simulink model "sampleModel2035"  (R2023a)
settings: Solver=VariableStepAuto  StartTime=0.0  StopTime=10.0  RelTol=1e-3
libraries: hdlsllib x11, simulink x2
settings Model: Creator=user1  LastModifiedBy=user1

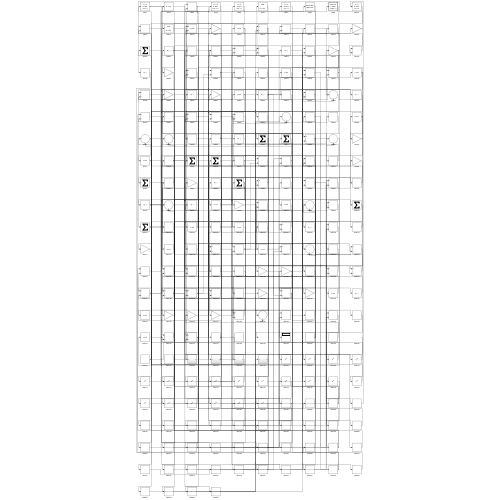
[thumbnail: Simulink's stored preview of the top-level diagram]
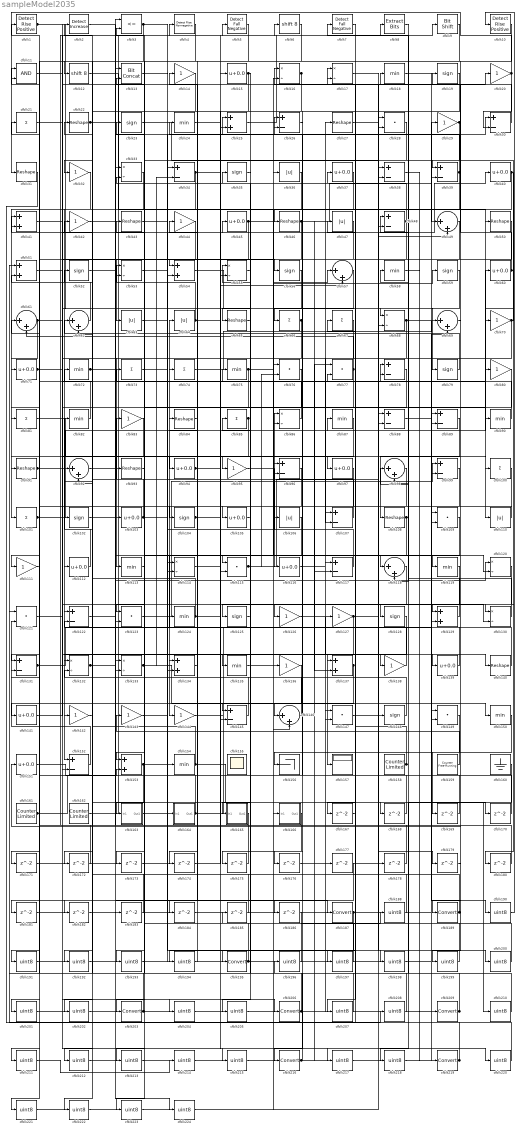
== system sampleModel2035 ==
  cfblk1 : hdlsllib/Logic and Bit Operations/Detect Rise Positive  vinit=0  OutDataTypeStr=boolean
  cfblk10 : hdlsllib/Logic and Bit Operations/Detect Rise Positive  vinit=0  OutDataTypeStr=boolean
  cfblk{21,66..67,73..74,81,85,100..101} (9 alike) : Sum  Inputs=+
  cfblk{19,23,35,52,56,59,79,102,104,125,128,148} (12 alike) : Signum
  cfblk{15,37,40,45,60,71,94,97,103,105,112,116,139,141,151} (15 alike) : Bias  Bias=0.0  SaturateOnIntegerOverflow=off
  cfblk{36,47,63..64,106,110} (6 alike) : Abs  SaturateOnIntegerOverflow=off
  cfblk{26,30,34,38..39,48,78,88..89,96,99,107,117,122,131,145,152} (17 alike) : Sum  Inputs=+-
  cfblk{22,27,31,43,46,50,65,84,91,93,108,140} (12 alike) : Reshape
  cfblk{28,76..77,109,115,121,123,147,149} (9 alike) : DotProduct  OutDataTypeStr=Inherit: Inherit via internal rule
  cfblk11 : Logic  AllPortsSameDT=off  OutDataTypeStr=boolean
  cfblk{14,20,29,32,42,44,70,80,83,95,111,126..127,136,138,142..144} (18 alike) : Gain
  cfblk{18,24,58,72,75,82,87,90,113,119,124,135,150,154} (14 alike) : MinMax
  cfblk{16..17,33,53,55,68,86,114,120,130,132..133} (12 alike) : Product  Inputs=*/  RndMeth=Zero  SaturateOnIntegerOverflow=on
  cfblk{49,57,61..62,69,92,98,118,146} (9 alike) : Sum  Inputs=|++
  cfblk12 : ArithShift  BitShiftNumber=8
  cfblk{25,41,51,54,129,134,137,153} (8 alike) : Sum
  cfblk13 : hdlsllib/Logic and Bit Operations/Bit Concat  numInputs=2
  cfblk155 : Scope
      settings: Floating=on
  cfblk156 : Terminator
  cfblk157 : Display
  cfblk158 : hdlsllib/Sources/Counter Limited  uplimit=7  tsamp=-1
  cfblk159 : hdlsllib/Sources/Counter Free-Running  NumBits=16  tsamp=-1
  cfblk160 : Ground
  cfblk161 : hdlsllib/Sources/Counter Limited  uplimit=7  tsamp=-1
  cfblk162 : hdlsllib/Sources/Counter Limited  uplimit=7  tsamp=-1
  cfblk163 : Subsystem
      settings: LibrarySourceBlock=|
      | hdlsllib/Ports &
      | Subsystems/Subsystem
  cfblk164 : Subsystem
      settings: LibrarySourceBlock=|
      | hdlsllib/Ports &
      | Subsystems/Subsystem
  cfblk165 : Subsystem
      settings: LibrarySourceBlock=|
      | hdlsllib/Ports &
      | Subsystems/Subsystem
  cfblk166 : Subsystem
      settings: LibrarySourceBlock=|
      | hdlsllib/Ports &
      | Subsystems/Subsystem
  cfblk{167..186} (20 alike) : Delay  SampleTime=1
  cfblk{187,189,195,203,206,209,216,219} (8 alike) : DataTypeConversion  SaturateOnIntegerOverflow=off  RndMeth=Floor
  cfblk{188,190..194,196..202,204..205,207..208,210..215,217..218,220..224} (30 alike) : DataTypeConversion  OutDataTypeStr=uint8  SaturateOnIntegerOverflow=off  RndMeth=Floor
  cfblk2 : simulink/Logic and Bit Operations/Detect Increase  vinit=0.0  OutDataTypeStr=boolean
      settings: LibrarySourceBlock=|
      | hdlsllib/Logic and Bit
      | Operations/Detect
      | Increase
  cfblk3 : RelationalOperator  Operator=<=  OutDataTypeStr=boolean  InputSameDT=off
  cfblk4 : hdlsllib/Logic and Bit Operations/Detect Rise Nonnegative  vinit=0  OutDataTypeStr=boolean
  cfblk5 : hdlsllib/Logic and Bit Operations/Detect Fall Negative  vinit=0  OutDataTypeStr=boolean
  cfblk6 : ArithShift  BitShiftNumber=8
  cfblk7 : hdlsllib/Logic and Bit Operations/Detect Fall Negative  vinit=0  OutDataTypeStr=boolean
  cfblk8 : simulink/Logic and Bit Operations/Extract Bits  bitsToExtract=Upper half  numBits=8  bitIdxRange=[0 7]  outScalingMode=Preserve fixed-point scaling
      settings: LibrarySourceBlock=|
      | hdlsllib/Logic and Bit
      | Operations/Extract Bits
  cfblk9 : hdlsllib/Logic and Bit Operations/Bit Shift  mode=Shift Left Logical  N=0
  wires:
  cfblk36/1 -> cfblk152/1
  cfblk117/1 -> cfblk86/1
  cfblk162/1 -> cfblk40/1
  cfblk165/1(Out1) -> cfblk4/1
  cfblk66/1 -> cfblk113/1, cfblk152/2
  cfblk72/1 -> cfblk5/1, cfblk119/1
  cfblk52/1 -> cfblk133/1
  cfblk118/1 -> cfblk128/1
  cfblk128/1 -> cfblk157/1
  cfblk103/1 -> cfblk83/1, cfblk130/2
  cfblk25/1 -> cfblk9/1
  cfblk75/1 -> cfblk123/1, cfblk57/1
  cfblk23/1 -> cfblk148/1
  cfblk124/1 -> cfblk92/2, cfblk217/1
  cfblk139/1 -> cfblk64/1
  cfblk59/1 -> cfblk79/1
  cfblk89/1 -> cfblk108/1
  cfblk123/1 -> cfblk99/1
  cfblk57/1 -> cfblk95/1
  cfblk20/1 -> cfblk31/1, cfblk30/2
  cfblk49/1 -> cfblk63/1
  cfblk1/1 -> cfblk68/1, cfblk68/2
  cfblk104/1 -> cfblk15/1, cfblk30/1
  cfblk13/1 -> cfblk164/1(In1)
  cfblk37/1 -> cfblk122/1
  cfblk38/1 -> cfblk219/1
  cfblk129/1 -> cfblk62/1
  cfblk146/1 -> cfblk52/1
  cfblk152/1 -> cfblk121/2
  cfblk86/1 -> cfblk43/1
  cfblk16/1 -> cfblk94/1, cfblk134/2
  cfblk142/1 -> cfblk42/1
  cfblk69/1 -> cfblk151/1
  cfblk32/1 -> cfblk101/1
  cfblk131/1 -> cfblk76/1, cfblk135/1
  cfblk2/1 -> cfblk187/1
  cfblk5/1 -> cfblk153/1
  cfblk26/1 -> cfblk46/1
  cfblk106/1 -> cfblk144/1
  cfblk42/1 -> cfblk19/1
  cfblk109/1 -> cfblk203/1
  cfblk10/1 -> cfblk189/1
  cfblk132/1 -> cfblk120/1, cfblk224/1
  cfblk100/1 -> cfblk142/1
  cfblk45/1 -> cfblk120/2, cfblk181/1
  cfblk154/1 -> cfblk92/1, cfblk210/1
  cfblk135/1 -> cfblk59/1
  cfblk107/1 -> cfblk41/1
  cfblk65/1 -> cfblk125/1
  cfblk164/1(Out1) -> cfblk89/1, cfblk21/1
  cfblk81/1 -> cfblk97/1
  cfblk40/1 -> cfblk86/2, cfblk70/1
  cfblk110/1 -> cfblk103/1
  cfblk77/1 -> cfblk126/1, cfblk61/2
  cfblk94/1 -> cfblk87/1, cfblk57/2
  cfblk30/1 -> cfblk16/1
  cfblk144/1 -> cfblk16/2
  cfblk121/1 -> cfblk18/1
  cfblk39/1 -> cfblk156/1, cfblk24/1
  cfblk41/1 -> cfblk56/1
  cfblk70/1 -> cfblk39/1, cfblk114/2
  cfblk15/1 -> cfblk65/1, cfblk55/2
  cfblk12/1 -> cfblk110/1
  cfblk137/1 -> cfblk132/2, cfblk223/1
  cfblk50/1 -> cfblk104/1
  cfblk83/1 -> cfblk112/1
  cfblk163/1(Out1) -> cfblk25/1
  cfblk105/1 -> cfblk145/1
  cfblk76/1 -> cfblk145/2
  cfblk35/1 -> cfblk115/1
  cfblk22/1 -> cfblk124/1, cfblk168/1
  cfblk112/1 -> cfblk82/1
  cfblk138/1 -> cfblk72/1
  cfblk97/1 -> cfblk146/1
  cfblk4/1 -> cfblk81/1
  cfblk108/1 -> cfblk163/1(In1), cfblk48/1
  cfblk99/1 -> cfblk141/1
  cfblk92/1 -> cfblk139/1
  cfblk47/1 -> cfblk91/1
  cfblk43/1 -> cfblk154/1
  cfblk90/1 -> cfblk23/1
  cfblk48/1 -> cfblk131/1, cfblk33/2
  cfblk151/1 -> cfblk153/2
  cfblk133/1 -> cfblk150/1, cfblk34/2
  cfblk9/1 -> cfblk54/1
  cfblk145/1 -> cfblk22/1
  cfblk85/1 -> cfblk171/1, cfblk172/1
  cfblk55/1 -> cfblk105/1
  cfblk74/1 -> cfblk39/2
  cfblk115/1 -> cfblk20/1, cfblk76/2
  cfblk80/1 -> cfblk118/1
  cfblk122/1 -> cfblk26/1
  cfblk60/1 -> cfblk17/1, cfblk130/1, cfblk180/1
  cfblk148/1 -> cfblk84/1
  cfblk8/1 -> cfblk118/2
  cfblk134/1 -> cfblk74/1
  cfblk71/1 -> cfblk111/1, cfblk90/1
  cfblk68/1 -> cfblk99/2, cfblk107/2
  cfblk24/1 -> cfblk6/1
  cfblk143/1 -> cfblk75/1
  cfblk46/1 -> cfblk29/1, cfblk137/2, cfblk50/1, cfblk184/1
  cfblk79/1 -> cfblk55/1
  cfblk3/1 -> cfblk69/1, cfblk32/1
  cfblk73/1 -> cfblk195/1
  cfblk101/1 -> cfblk60/1, cfblk45/1
  cfblk140/1 -> cfblk85/1
  cfblk56/1 -> cfblk66/1
  cfblk14/1 -> cfblk132/1
  cfblk153/1 -> cfblk106/1, cfblk192/1
  cfblk125/1 -> cfblk165/1(In1)
  cfblk58/1 -> cfblk209/1
  cfblk33/1 -> cfblk123/2
  cfblk53/1 -> cfblk114/1
  cfblk158/1 -> cfblk67/1, cfblk78/1, cfblk78/2
  cfblk113/1 -> cfblk53/1
  cfblk149/1 -> cfblk216/1
  cfblk161/1 -> cfblk133/2, cfblk11/2
  cfblk127/1 -> cfblk49/2, cfblk182/1
  cfblk34/1 -> cfblk129/1, cfblk221/1
  cfblk29/1 -> cfblk48/2, cfblk167/1
  cfblk62/1 -> cfblk11/1
  cfblk61/1 -> cfblk71/1, cfblk8/1
  cfblk126/1 -> cfblk140/1
  cfblk91/1 -> cfblk33/1, cfblk100/1, cfblk129/2
  cfblk6/1 -> cfblk12/1
  cfblk95/1 -> cfblk116/1
  cfblk78/1 -> cfblk134/1
  cfblk64/1 -> cfblk3/2, cfblk138/1
  cfblk159/1 -> cfblk143/1
  cfblk18/1 -> cfblk49/1
  cfblk82/1 -> cfblk61/1
  cfblk116/1 -> cfblk27/1
  cfblk141/1 -> cfblk80/1
  cfblk130/1 -> cfblk7/1
  cfblk54/1 -> cfblk88/2
  cfblk51/1 -> cfblk206/1
  cfblk7/1 -> cfblk137/1
  cfblk168/1 -> cfblk117/1
  cfblk150/1 -> cfblk169/1
  cfblk169/1 -> cfblk26/2
  cfblk63/1 -> cfblk170/1
  cfblk170/1 -> cfblk13/1
  cfblk171/1 -> cfblk25/2
  cfblk172/1 -> cfblk1/1
  cfblk93/1 -> cfblk173/1
  cfblk173/1 -> cfblk115/2
  cfblk84/1 -> cfblk174/1
  cfblk166/1(Out1) -> cfblk175/1
  cfblk175/1 -> cfblk41/2
  cfblk120/1 -> cfblk176/1
  cfblk176/1 -> cfblk88/1
  cfblk27/1 -> cfblk178/1
  cfblk178/1 -> cfblk3/1
  cfblk17/1 -> cfblk179/1
  cfblk180/1 -> cfblk131/2
  cfblk181/1 -> cfblk54/2
  cfblk182/1 -> cfblk107/1
  cfblk102/1 -> cfblk183/1
  cfblk183/1 -> cfblk122/2
  cfblk184/1 -> cfblk89/2
  cfblk185/1 -> cfblk53/2
  cfblk19/1 -> cfblk186/1
  cfblk187/1 -> cfblk47/1, cfblk194/1
  cfblk186/1 -> cfblk188/1
  cfblk188/1 -> cfblk2/1
  cfblk189/1 -> cfblk17/2, cfblk37/1
  cfblk88/1 -> cfblk190/1
  cfblk190/1 -> cfblk10/1
  cfblk177/1 -> cfblk191/1
  cfblk191/1 -> cfblk69/2
  cfblk192/1 -> cfblk177/1
  cfblk44/1 -> cfblk193/1
  cfblk193/1 -> cfblk34/1
  cfblk194/1 -> cfblk44/1
  cfblk195/1 -> cfblk14/1, cfblk146/2
  cfblk196/1 -> cfblk73/1
  cfblk98/1 -> cfblk197/1
  cfblk197/1 -> cfblk35/1
  cfblk114/1 -> cfblk198/1
  cfblk198/1 -> cfblk98/1
  cfblk179/1 -> cfblk199/1
  cfblk199/1 -> cfblk98/2
  cfblk147/1 -> cfblk200/1
  cfblk200/1 -> cfblk93/1
  cfblk111/1 -> cfblk201/1
  cfblk201/1 -> cfblk147/1
  cfblk67/1 -> cfblk202/1
  cfblk202/1 -> cfblk147/2
  cfblk203/1 -> cfblk102/1, cfblk127/1
  cfblk21/1 -> cfblk204/1
  cfblk204/1 -> cfblk109/1
  cfblk119/1 -> cfblk205/1
  cfblk205/1 -> cfblk109/2
  cfblk206/1 -> cfblk62/2, cfblk117/2
  cfblk167/1 -> cfblk207/1
  cfblk207/1 -> cfblk51/1
  cfblk31/1 -> cfblk208/1
  cfblk208/1 -> cfblk51/2
  cfblk209/1 -> cfblk185/1, cfblk13/2
  cfblk210/1 -> cfblk58/1
  cfblk136/1 -> cfblk211/1
  cfblk87/1 -> cfblk212/1
  cfblk212/1 -> cfblk136/1
  cfblk28/1 -> cfblk213/1
  cfblk213/1 -> cfblk166/1(In1)
  cfblk211/1 -> cfblk214/1
  cfblk214/1 -> cfblk28/1
  cfblk11/1 -> cfblk215/1
  cfblk215/1 -> cfblk28/2
  cfblk216/1 -> cfblk196/1, cfblk77/1
  cfblk217/1 -> cfblk149/1
  cfblk160/1 -> cfblk218/1
  cfblk218/1 -> cfblk149/2
  cfblk219/1 -> cfblk77/2, cfblk121/1
  cfblk174/1 -> cfblk220/1
  cfblk220/1 -> cfblk38/1
  cfblk221/1 -> cfblk38/2
  cfblk96/1 -> cfblk222/1
  cfblk222/1 -> cfblk36/1
  cfblk223/1 -> cfblk96/1
  cfblk224/1 -> cfblk96/2

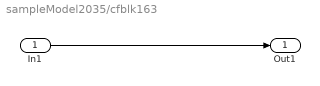
== system sampleModel2035/cfblk163 ==
  In1 : Inport
  Out1 : Outport
  wires:
  In1/1 -> Out1/1

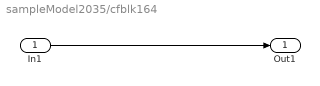
== system sampleModel2035/cfblk164 ==
  In1 : Inport
  Out1 : Outport
  wires:
  In1/1 -> Out1/1

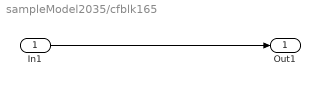
== system sampleModel2035/cfblk165 ==
  In1 : Inport
  Out1 : Outport
  wires:
  In1/1 -> Out1/1

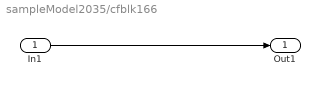
== system sampleModel2035/cfblk166 ==
  In1 : Inport
  Out1 : Outport
  wires:
  In1/1 -> Out1/1
